simulink model "Microgrid_with_3VOCs"  (R2018a)
settings: Solver=VariableStepAuto  StartTime=0.0  StopTime=1  FixedStep=1e-4  MaxStep=1e-4  RelTol=1e-3
values from neighbouring files (symbols this model uses):
  Cosc = (P * Qf) / (wosc * Vrms^2)    [EpsilonGrapher.m]
  del = dK * Vrms * sqrt(2)    [EpsilonGrapher.m]
  k = double(Ms / zsysSupr)    [EpsilonGrapher.m]
  Lnet = (Vrms^2 * Lnpu) / (P * wosc)    (= 0.0198943678865)    [EpsilonGrapher.m]
  Losc = Vrms^2 / (wosc * P * Qf)    [EpsilonGrapher.m]
  Rnet = (Vrms^2 * Rnpu) / P    (= 6.25)    [EpsilonGrapher.m]
  Rosc = Vrms^2 / P    (= 62.5)    [EpsilonGrapher.m]
  Vrms = 250    [EpsilonGrapher.m]
undefined symbols (not defined in the file or in its folder): A, Continuous, fosc, gcbh, LIBRARY__Improved_VoC_with_DFs__2018_04_03__0, sps, sps_rtmsupport, spsMeanValueVariableFrequencyModel, spsPLLModel, VoC
libraries: powerlib x28, powerlib_meascontrol x13
settings Model: Creator=University  LastModifiedBy=rbtmc
settings SolverCC: ZeroCrossAlgorithm=Adaptive
settings DebuggingCC: MaxConsecutiveZCsMsg=none
settings CodeAppCC: StateflowObjectComments=on
settings SimscapeCC: SimscapeNormalizeSystem=off

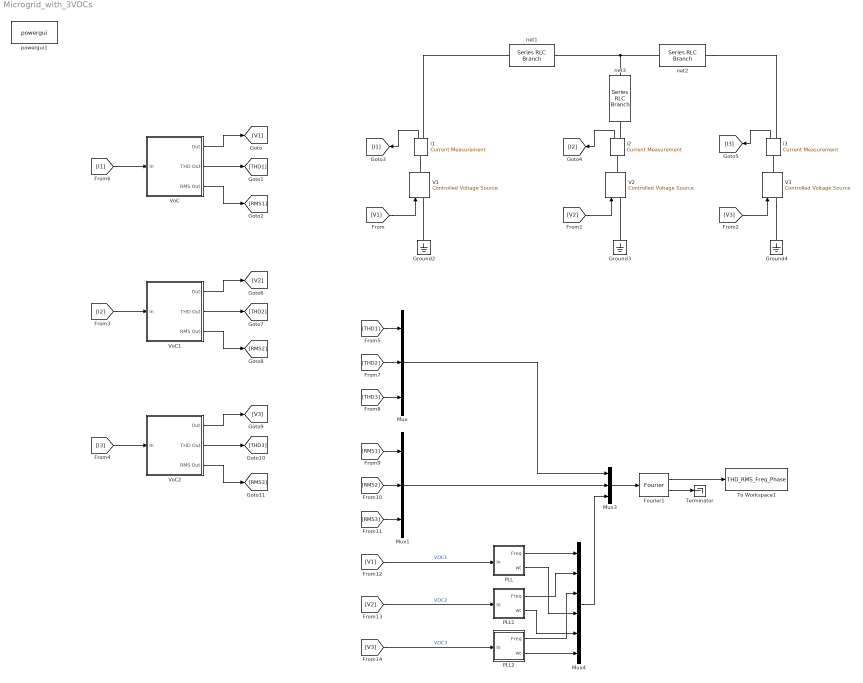
== system Microgrid_with_3VOCs ==
  Fourier1 : powerlib_meascontrol/Measurements/Fourier  Freq=50  n=0  InInit=[0, 0]  Ts=0
      settings: SourceProductName=Simscape Power Systems
  Ground2 : powerlib/Elements/Ground  LConnTagsString=a
  Ground3 : powerlib/Elements/Ground  LConnTagsString=a
  Ground4 : powerlib/Elements/Ground  LConnTagsString=a
  Mux : Mux  Inputs=3
  Mux1 : Mux  Inputs=3
  Mux3 : Mux  Inputs=3
  Mux4 : Mux  Inputs=6
  PLL : Subsystem  AncestorBlock=powerlib_meascontrol/PLL/PLL  DialogController=POWERSYS.PowerSysDialog  LoadFcn=sps_rtmsupport('LoadFcn', gcbh);  StartFcn=sps_rtmsupport('StartFcn', gcbh);  StopFcn=sps_rtmsupport('StopFcn', gcbh);  mask(PLL){Fmin=45, Par_Init=[0, 50], ParK=[180, 3200, 1], TcD=1e-4, MaxRateChangeFreq=12, FilterCutOffFreq=25, Ts=0, AGC=off}
      mask prompts: Fmin "Minimum frequency (Hz):"; Par_Init "Initial inputs [ Phase (degrees), Frequency (Hz) ]:"; ParK "Regulator gains [ Kp, Ki, Kd ]:"; TcD "Time constant for derivative action (s):"; MaxRateChangeFreq "Maximum rate of change of frequency (Hz/s):"; FilterCutOffFreq "Filter cut-off frequency for frequency measurement (Hz):"; Ts "Sample time:"; AGC "Enable automatic gain control"
      mask help:
      | This Phase Locked Loop (PLL) system can be used  to synchronize on a variable frequency sinusoidal signal. When the Automatic Gain Control is enabled, the input (phase error) of the PLL regulator is scaled according to the input signal magnitude.
      |
      | For optimal performance, set regulator gains [ Kp Ki  Kd ] = [ 180  3200  1 ] and check the Enable Automatic Gain Control parameter.
      |
      | Input : Normalized input signal (pu)
      | Output 1:  Measured frequency (Hz) = w/(2pi)
      | Output 2:  Ramp w.t varying between 0 and 2*pi, synchronized on the zero-crossing (rising) of the fundamental of input signal.
      mask init:
      | block=gcb;
      | [WantBlockChoice,Ts,sps] = powericon('PLLInit',block,Fmin,Par_Init,ParK,TcD,MaxRateChangeFreq,FilterCutOffFreq,AGC,Ts);
      | powericon('SetInternalModels','set',block,WantBlockChoice);
      settings: CopyFcn=sps_rtmsupport('CopyFcn', gcbh);  DeleteFcn=sps_rtmsupport('DeleteFcn', gcbh);  UndoDeleteFcn=sps_rtmsupport('UndoDeleteFcn', gcbh);  ModelCloseFcn=sps_rtmsupport('ModelCloseFcn', gcbh);  PreSaveFcn=sps_rtmsupport('PreSaveFcn', gcbh);  PostSaveFcn=sps_rtmsupport('PostSaveFcn', gcbh);  NameChangeFcn=sps_rtmsupport('NameChangeFcn', gcbh);  PreCopyFcn=sps_rtmsupport('PreCopyFcn', gcbh);  OpenFcn=sps_rtmsupport('OpenFcn', gcbh, [8]);  CloseFcn=sps_rtmsupport('CloseFcn', gcbh);  PreDeleteFcn=sps_rtmsupport('PreDeleteFcn', gcbh);
      mask Help: helpview(psbhelp);
  PLL1 : Subsystem  AncestorBlock=powerlib_meascontrol/PLL/PLL  DialogController=POWERSYS.PowerSysDialog  LoadFcn=sps_rtmsupport('LoadFcn', gcbh);  StartFcn=sps_rtmsupport('StartFcn', gcbh);  StopFcn=sps_rtmsupport('StopFcn', gcbh);  mask(PLL){Fmin=45, Par_Init=[0, 50], ParK=[180, 3200, 1], TcD=1e-4, MaxRateChangeFreq=12, FilterCutOffFreq=25, Ts=0, AGC=off}
      mask prompts: Fmin "Minimum frequency (Hz):"; Par_Init "Initial inputs [ Phase (degrees), Frequency (Hz) ]:"; ParK "Regulator gains [ Kp, Ki, Kd ]:"; TcD "Time constant for derivative action (s):"; MaxRateChangeFreq "Maximum rate of change of frequency (Hz/s):"; FilterCutOffFreq "Filter cut-off frequency for frequency measurement (Hz):"; Ts "Sample time:"; AGC "Enable automatic gain control"
      mask help:
      | This Phase Locked Loop (PLL) system can be used  to synchronize on a variable frequency sinusoidal signal. When the Automatic Gain Control is enabled, the input (phase error) of the PLL regulator is scaled according to the input signal magnitude.
      |
      | For optimal performance, set regulator gains [ Kp Ki  Kd ] = [ 180  3200  1 ] and check the Enable Automatic Gain Control parameter.
      |
      | Input : Normalized input signal (pu)
      | Output 1:  Measured frequency (Hz) = w/(2pi)
      | Output 2:  Ramp w.t varying between 0 and 2*pi, synchronized on the zero-crossing (rising) of the fundamental of input signal.
      mask init:
      | block=gcb;
      | [WantBlockChoice,Ts,sps] = powericon('PLLInit',block,Fmin,Par_Init,ParK,TcD,MaxRateChangeFreq,FilterCutOffFreq,AGC,Ts);
      | powericon('SetInternalModels','set',block,WantBlockChoice);
      settings: CopyFcn=sps_rtmsupport('CopyFcn', gcbh);  DeleteFcn=sps_rtmsupport('DeleteFcn', gcbh);  UndoDeleteFcn=sps_rtmsupport('UndoDeleteFcn', gcbh);  ModelCloseFcn=sps_rtmsupport('ModelCloseFcn', gcbh);  PreSaveFcn=sps_rtmsupport('PreSaveFcn', gcbh);  PostSaveFcn=sps_rtmsupport('PostSaveFcn', gcbh);  NameChangeFcn=sps_rtmsupport('NameChangeFcn', gcbh);  PreCopyFcn=sps_rtmsupport('PreCopyFcn', gcbh);  OpenFcn=sps_rtmsupport('OpenFcn', gcbh, [8]);  CloseFcn=sps_rtmsupport('CloseFcn', gcbh);  PreDeleteFcn=sps_rtmsupport('PreDeleteFcn', gcbh);
      mask Help: helpview(psbhelp);
  PLL2 : Subsystem  AncestorBlock=powerlib_meascontrol/PLL/PLL  DialogController=POWERSYS.PowerSysDialog  LoadFcn=sps_rtmsupport('LoadFcn', gcbh);  StartFcn=sps_rtmsupport('StartFcn', gcbh);  StopFcn=sps_rtmsupport('StopFcn', gcbh);  mask(PLL){Fmin=45, Par_Init=[0, 50], ParK=[180, 3200, 1], TcD=1e-4, MaxRateChangeFreq=12, FilterCutOffFreq=25, Ts=0, AGC=off}
      mask prompts: Fmin "Minimum frequency (Hz):"; Par_Init "Initial inputs [ Phase (degrees), Frequency (Hz) ]:"; ParK "Regulator gains [ Kp, Ki, Kd ]:"; TcD "Time constant for derivative action (s):"; MaxRateChangeFreq "Maximum rate of change of frequency (Hz/s):"; FilterCutOffFreq "Filter cut-off frequency for frequency measurement (Hz):"; Ts "Sample time:"; AGC "Enable automatic gain control"
      mask help:
      | This Phase Locked Loop (PLL) system can be used  to synchronize on a variable frequency sinusoidal signal. When the Automatic Gain Control is enabled, the input (phase error) of the PLL regulator is scaled according to the input signal magnitude.
      |
      | For optimal performance, set regulator gains [ Kp Ki  Kd ] = [ 180  3200  1 ] and check the Enable Automatic Gain Control parameter.
      |
      | Input : Normalized input signal (pu)
      | Output 1:  Measured frequency (Hz) = w/(2pi)
      | Output 2:  Ramp w.t varying between 0 and 2*pi, synchronized on the zero-crossing (rising) of the fundamental of input signal.
      mask init:
      | block=gcb;
      | [WantBlockChoice,Ts,sps] = powericon('PLLInit',block,Fmin,Par_Init,ParK,TcD,MaxRateChangeFreq,FilterCutOffFreq,AGC,Ts);
      | powericon('SetInternalModels','set',block,WantBlockChoice);
      settings: CopyFcn=sps_rtmsupport('CopyFcn', gcbh);  DeleteFcn=sps_rtmsupport('DeleteFcn', gcbh);  UndoDeleteFcn=sps_rtmsupport('UndoDeleteFcn', gcbh);  ModelCloseFcn=sps_rtmsupport('ModelCloseFcn', gcbh);  PreSaveFcn=sps_rtmsupport('PreSaveFcn', gcbh);  PostSaveFcn=sps_rtmsupport('PostSaveFcn', gcbh);  NameChangeFcn=sps_rtmsupport('NameChangeFcn', gcbh);  PreCopyFcn=sps_rtmsupport('PreCopyFcn', gcbh);  OpenFcn=sps_rtmsupport('OpenFcn', gcbh, [8]);  CloseFcn=sps_rtmsupport('CloseFcn', gcbh);  PreDeleteFcn=sps_rtmsupport('PreDeleteFcn', gcbh);
      mask Help: helpview(psbhelp);
  Terminator : Terminator
  To Workspace1 : ToWorkspace  VariableName=THD_RMS_Freq_Phase  SampleTime=-1
      settings: MaxDataPoints=1
  V1 : powerlib/Electrical Sources/Controlled Voltage Source  Initialize=off  Source_Type=AC  Amplitude=A  Phase=0  Frequency=fosc  Measurements=None
  V2 : powerlib/Electrical Sources/Controlled Voltage Source  Initialize=off  Source_Type=AC  Amplitude=A  Phase=120  Frequency=fosc  Measurements=None
  V3 : powerlib/Electrical Sources/Controlled Voltage Source  Initialize=off  Source_Type=AC  Amplitude=A  Phase=240  Frequency=fosc  Measurements=None
  VoC : Subsystem  AncestorBlock=LIBRARY__Improved_VoC_with_DFs__2018_04_03__0/VoC
  VoC1 : Subsystem  AncestorBlock=LIBRARY__Improved_VoC_with_DFs__2018_04_03__0/VoC
  VoC2 : Subsystem  AncestorBlock=LIBRARY__Improved_VoC_with_DFs__2018_04_03__0/VoC
  i1 : powerlib/Measurements/Current Measurement  PhasorSimulation=off  OutputType=Complex  PSBequivalent=0
  i2 : powerlib/Measurements/Current Measurement  PhasorSimulation=off  OutputType=Complex  PSBequivalent=0
  i3 : powerlib/Measurements/Current Measurement  PhasorSimulation=off  OutputType=Complex  PSBequivalent=0
  net1 : powerlib/Elements/Series RLC Branch  LConnTagsString=__new0  RConnTagsString=__new0  BranchType=RL  Resistance=Rnet  Inductance=Lnet  SetiL0=off  InitialCurrent=0  Capacitance=16.2e-3  Setx0=off  InitialVoltage=0  Measurements=None
  net2 : powerlib/Elements/Series RLC Branch  LConnTagsString=__new0  RConnTagsString=__new0  BranchType=RL  Resistance=Rnet  Inductance=Lnet  SetiL0=off  InitialCurrent=0  Capacitance=16.2e-3  Setx0=off  InitialVoltage=0  Measurements=None
  net3 : powerlib/Elements/Series RLC Branch  LConnTagsString=__new0  RConnTagsString=__new0  BranchType=RL  Resistance=Rnet  Inductance=Lnet  SetiL0=off  InitialCurrent=0  Capacitance=16.2e-3  Setx0=off  InitialVoltage=0  Measurements=None
  powergui1 : powerlib/powergui  Priority=1  SimulationMode=Discrete  SampleTime=50e-6  frequency=60  Iterations=50  frequencyindice=0  Pbase=100e6  ErrMax=1e-4  UnitsV=kV  UnitsW=MW  buscounter=0  FunctionMessages=off  echomessages=off  EnableUseOfTLC=off  CurrentSourceSwitches=off  DisableSnubberDevices=off  DisableRonSwitches=off  DisableVfSwitches=off  DisplayEquations=off  SolverType=Tustin/Backward Euler (TBE)  Interpol=off  ExternalGateDelay=off  methode=off  Ts=100  x0status=blocks  SPID=off  SwTol=0  HookPort=off  RestoreLinks=warning  ResistiveCurrentMeasurement=off  Frange=[0:2:500]  Ylog=off  Xlog=on  ShowGrid=off  save=off  variable=ZData  structure=0  ZoomFFT=off  StartTime=0.0  cycles=1  DisplayStyle=1  fundamental=60  FreqAxis=off  MaxFrequency=1000  frequencyindicesteady=1  RmsSteady=1  display=off
  wires:
  VoC/1(Out) -> [V1]
  VoC/2(THD Out) -> [THD1]
  VoC/3(RMS Out) -> [RMS1]
  [I1] -> VoC/1(In)
  i3/1 -> [I3]
  [V1] -> V1/1
  [V3] -> V3/1
  i2/1 -> [I2]
  i1/1 -> [I1]
  [V2] -> V2/1
  [I2] -> VoC1/1(In)
  VoC1/1(Out) -> [V2]
  VoC1/3(RMS Out) -> [RMS2]
  VoC1/2(THD Out) -> [THD2]
  [I3] -> VoC2/1(In)
  VoC2/1(Out) -> [V3]
  VoC2/3(RMS Out) -> [RMS3]
  VoC2/2(THD Out) -> [THD3]
  [THD1] -> Mux/1
  [THD2] -> Mux/2
  [THD3] -> Mux/3
  [RMS1] -> Mux1/1
  [RMS3] -> Mux1/3
  [RMS2] -> Mux1/2
  Mux/1 -> Mux3/1
  Mux1/1 -> Mux3/2
  [V1] -> PLL/1(In)  "VOC1"
  [V2] -> PLL1/1(In)  "VOC2"
  [V3] -> PLL2/1(In)  "VOC3"
  Mux3/1 -> Fourier1/1
  PLL/1(Freq) -> Mux4/1
  PLL1/1(Freq) -> Mux4/2
  PLL2/1(Freq) -> Mux4/3
  Mux4/1 -> Mux3/3
  Fourier1/1 -> To Workspace1/1
  PLL/2(wt) -> Mux4/4
  PLL1/2(wt) -> Mux4/5
  PLL2/2(wt) -> Mux4/6
  Fourier1/2 -> Terminator/1
  connections:
  i2/RConn1 -- net3/RConn1
  net1/RConn1 -- i1/RConn1
  i1/LConn1 -- V1/RConn1
  net2/RConn1 -- i3/RConn1
  V2/RConn1 -- i2/LConn1
  V3/LConn1 -- Ground4/LConn1
  V2/LConn1 -- Ground3/LConn1
  V3/RConn1 -- i3/LConn1
  Ground2/LConn1 -- V1/LConn1
  net3/LConn1 -- net2/LConn1 -- net1/LConn1

== system Microgrid_with_3VOCs/PLL ==
  In : Inport  SampleTime=Ts
  Model : Subsystem  AncestorBlock=spsPLLModel/Continuous  DialogController=POWERSYS.PowerSysDialog
  Freq : Outport  SampleTime=Ts
  wt : Outport  Port=2  SampleTime=Ts
  wires:
  Model/2(wt) -> wt/1
  Model/1(Freq) -> Freq/1
  In/1 -> Model/1(In)

== system Microgrid_with_3VOCs/PLL1 ==
  In : Inport  SampleTime=Ts
  Model : Subsystem  AncestorBlock=spsPLLModel/Continuous  DialogController=POWERSYS.PowerSysDialog
  Freq : Outport  SampleTime=Ts
  wt : Outport  Port=2  SampleTime=Ts
  wires:
  Model/2(wt) -> wt/1
  Model/1(Freq) -> Freq/1
  In/1 -> Model/1(In)

== system Microgrid_with_3VOCs/PLL2 ==
  In : Inport  SampleTime=Ts
  Model : Subsystem  AncestorBlock=spsPLLModel/Continuous  DialogController=POWERSYS.PowerSysDialog
  Freq : Outport  SampleTime=Ts
  wt : Outport  Port=2  SampleTime=Ts
  wires:
  Model/2(wt) -> wt/1
  Model/1(Freq) -> Freq/1
  In/1 -> Model/1(In)

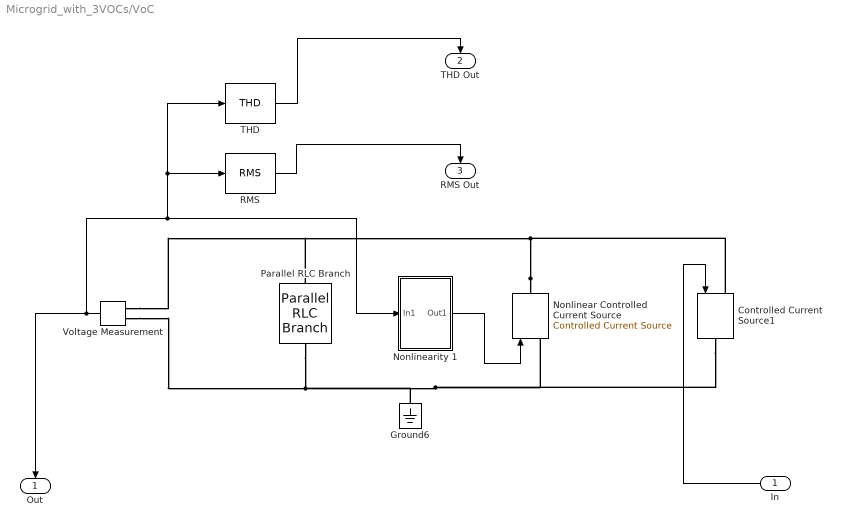
== system Microgrid_with_3VOCs/VoC ==
  In : Inport
  Controlled Current Source1 : powerlib/Electrical Sources/Controlled Current Source  Initialize=on  Source_Type=AC  Amplitude=0  Phase=0  Frequency=0  Measurements=None
  Ground6 : powerlib/Elements/Ground  LConnTagsString=a
  Nonlinear Controlled Current Source : powerlib/Electrical Sources/Controlled Current Source  Initialize=on  Source_Type=AC  Amplitude=0  Phase=0  Frequency=0  Measurements=None
  Nonlinearity 1 : Subsystem
  Parallel RLC Branch : powerlib/Elements/Parallel RLC Branch  LConnTagsString=a  RConnTagsString=__new0  BranchType=RLC  Resistance=Rosc  Inductance=Losc  SetiL0=off  InitialCurrent=0  Capacitance=Cosc  Setx0=on  InitialVoltage=Vrms * sqrt(2) * sind(0)  Measurements=None
  RMS : powerlib_meascontrol/Measurements/RMS  TrueRMS=on  Freq=50  RMSInit=0  Ts=0
  THD : powerlib_meascontrol/Measurements/THD  Freq=50  Ts=0
  Voltage Measurement : powerlib/Measurements/Voltage Measurement  PhasorSimulation=off  OutputType=Complex  PSBequivalent=0
  Out : Outport
  THD Out : Outport  Port=2
  RMS Out : Outport  Port=3
  wires:
  Voltage Measurement/1 -> THD/1, RMS/1, Nonlinearity 1/1(In1), Out/1
  In/1 -> Controlled Current Source1/1
  THD/1 -> THD Out/1
  RMS/1 -> RMS Out/1
  Nonlinearity 1/1(Out1) -> Nonlinear Controlled Current Source/1
  connections:
  Voltage Measurement/LConn2 -- Nonlinear Controlled Current Source/LConn1 -- Controlled Current Source1/RConn1 -- Ground6/LConn1 -- Parallel RLC Branch/RConn1
  Nonlinear Controlled Current Source/RConn1 -- Controlled Current Source1/LConn1 -- Voltage Measurement/LConn1 -- Parallel RLC Branch/LConn1

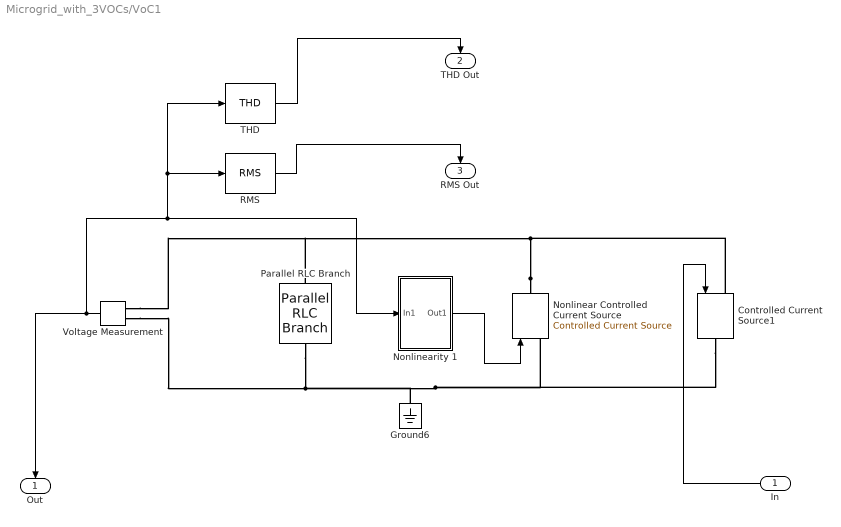
== system Microgrid_with_3VOCs/VoC1 ==
  In : Inport
  Controlled Current Source1 : powerlib/Electrical Sources/Controlled Current Source  Initialize=on  Source_Type=AC  Amplitude=0  Phase=0  Frequency=0  Measurements=None
  Ground6 : powerlib/Elements/Ground  LConnTagsString=a
  Nonlinear Controlled Current Source : powerlib/Electrical Sources/Controlled Current Source  Initialize=on  Source_Type=AC  Amplitude=0  Phase=0  Frequency=0  Measurements=None
  Nonlinearity 1 : Subsystem
  Parallel RLC Branch : powerlib/Elements/Parallel RLC Branch  LConnTagsString=a  RConnTagsString=__new0  BranchType=RLC  Resistance=Rosc  Inductance=Losc  SetiL0=off  InitialCurrent=0  Capacitance=Cosc  Setx0=on  InitialVoltage=Vrms * sqrt(2) * sind(45)  Measurements=None
  RMS : powerlib_meascontrol/Measurements/RMS  TrueRMS=on  Freq=50  RMSInit=0  Ts=0
  THD : powerlib_meascontrol/Measurements/THD  Freq=50  Ts=0
  Voltage Measurement : powerlib/Measurements/Voltage Measurement  PhasorSimulation=off  OutputType=Complex  PSBequivalent=0
  Out : Outport
  THD Out : Outport  Port=2
  RMS Out : Outport  Port=3
  wires:
  Voltage Measurement/1 -> THD/1, RMS/1, Nonlinearity 1/1(In1), Out/1
  In/1 -> Controlled Current Source1/1
  THD/1 -> THD Out/1
  RMS/1 -> RMS Out/1
  Nonlinearity 1/1(Out1) -> Nonlinear Controlled Current Source/1
  connections:
  Voltage Measurement/LConn2 -- Nonlinear Controlled Current Source/LConn1 -- Controlled Current Source1/RConn1 -- Ground6/LConn1 -- Parallel RLC Branch/RConn1
  Nonlinear Controlled Current Source/RConn1 -- Controlled Current Source1/LConn1 -- Voltage Measurement/LConn1 -- Parallel RLC Branch/LConn1

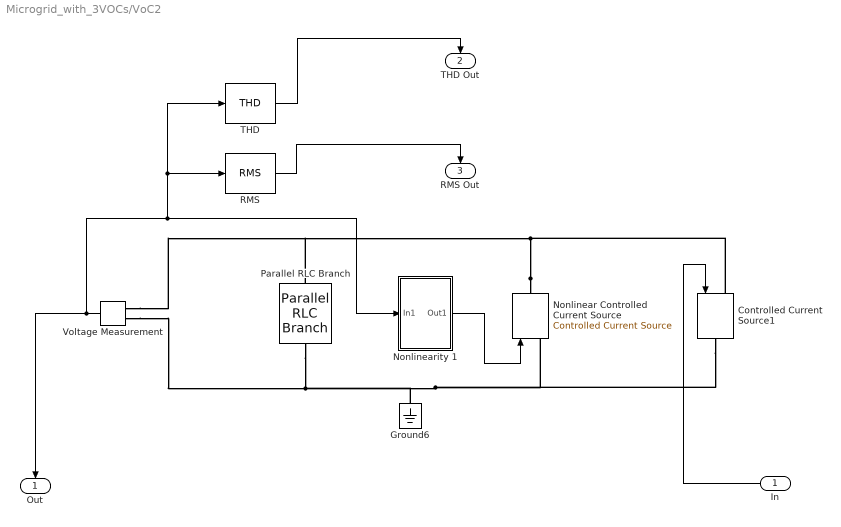
== system Microgrid_with_3VOCs/VoC2 ==
  In : Inport
  Controlled Current Source1 : powerlib/Electrical Sources/Controlled Current Source  Initialize=on  Source_Type=AC  Amplitude=0  Phase=0  Frequency=0  Measurements=None
  Ground6 : powerlib/Elements/Ground  LConnTagsString=a
  Nonlinear Controlled Current Source : powerlib/Electrical Sources/Controlled Current Source  Initialize=on  Source_Type=AC  Amplitude=0  Phase=0  Frequency=0  Measurements=None
  Nonlinearity 1 : Subsystem
  Parallel RLC Branch : powerlib/Elements/Parallel RLC Branch  LConnTagsString=a  RConnTagsString=__new0  BranchType=RLC  Resistance=Rosc  Inductance=Losc  SetiL0=off  InitialCurrent=0  Capacitance=Cosc  Setx0=on  InitialVoltage=Vrms * sqrt(2) * sind(90)  Measurements=None
  RMS : powerlib_meascontrol/Measurements/RMS  TrueRMS=on  Freq=50  RMSInit=0  Ts=0
  THD : powerlib_meascontrol/Measurements/THD  Freq=50  Ts=0
  Voltage Measurement : powerlib/Measurements/Voltage Measurement  PhasorSimulation=off  OutputType=Complex  PSBequivalent=0
  Out : Outport
  THD Out : Outport  Port=2
  RMS Out : Outport  Port=3
  wires:
  Voltage Measurement/1 -> THD/1, RMS/1, Nonlinearity 1/1(In1), Out/1
  In/1 -> Controlled Current Source1/1
  THD/1 -> THD Out/1
  RMS/1 -> RMS Out/1
  Nonlinearity 1/1(Out1) -> Nonlinear Controlled Current Source/1
  connections:
  Voltage Measurement/LConn2 -- Nonlinear Controlled Current Source/LConn1 -- Controlled Current Source1/RConn1 -- Ground6/LConn1 -- Parallel RLC Branch/RConn1
  Nonlinear Controlled Current Source/RConn1 -- Controlled Current Source1/LConn1 -- Voltage Measurement/LConn1 -- Parallel RLC Branch/LConn1

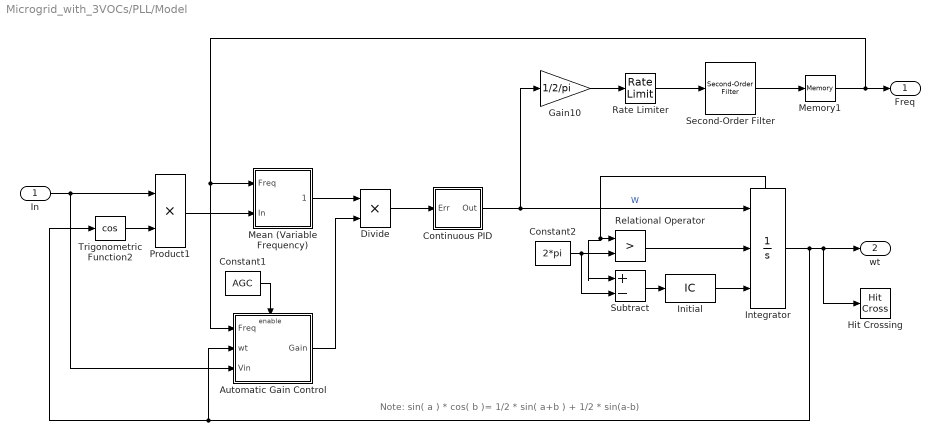
== system Microgrid_with_3VOCs/PLL/Model ==
  note: Note: sin( a ) * cos( b )= 1/2 * sin( a+b ) + 1/2 * sin(a-b)
  In : Inport
  Automatic Gain Control : Subsystem
  Constant1 : Constant  Value=AGC
  Constant2 : Constant  Value=2*pi
  Continuous PID : Subsystem  DialogController=POWERSYS.PowerSysDialog  VariantControl=PID_Continuous  mask(Continuous PID Controller){Kp=sps.Kp, Ki=sps.Ki, Kd=sps.Kd, TcD=sps.TcD, Par_Limits=[ inf  0 ], Init=2*pi*sps.Finit}
      mask prompts: Kp "Proportional gain (Kp):"; Ki "Integral gain (Ki):"; Kd "Derivative gain (Kd):"; TcD "Time constant for derivative filter (s):"; Par_Limits "Output limits: [ Upper   Lower ]"; Init "Output initial value:"
      mask help: This block implements a continuous PID controller.
      mask Display: disp('PID');
  Divide : Product
  Gain10 : Gain  Gain=1/2/pi  SaturateOnIntegerOverflow=on  OutDataTypeStr=Inherit: Same as input  ParamDataTypeStr=Inherit: Same as input
  Hit Crossing : HitCross  HitCrossingOffset=pi  HitCrossingDirection=falling  ShowOutputPort=off
  Initial : InitialCondition  Value=0
  Integrator : Integrator  ExternalReset=rising  InitialConditionSource=external  InitialCondition=sps.Phase_Init*pi/180  ShowStatePort=on
  Mean (Variable Frequency) : Subsystem  AncestorBlock=|  DialogController=POWERSYS.PowerSysDialog  LoadFcn=sps_rtmsupport('LoadFcn', gcbh);  StartFcn=sps_rtmsupport('StartFcn', gcbh);  StopFcn=sps_rtmsupport('StopFcn', gcbh);  mask(Mean (Variable Frequency)){Finit=sps.Finit, Fmin=sps.Fmin, Vinit=0, Ts=0}
      | powerlib_meascontrol/Measurements/Mean
      | (Variable Frequency)
      mask prompts: Finit "Initial frequency (Hz):"; Fmin "Minimum frequency (Hz):"; Vinit "Initial input (DC component):"; Ts "Sample time:"
      mask help:
      | Compute the mean value of input 2 over a running window of one cycle of frequency signal given by input 1.
      |
      | For the first cycle of initial frequency, the output is held to the value specified in the Initial input (DC component) parameter.
      |
      | The Minimum frequency parameter is used to determine the buffer size of the Variable Time Delay block used under the mask of the block.
      mask init:
      | block=gcb;
      | [WantBlockChoice,Ts,sps] = powericon('MeanVariableFrequencyInit',block,Finit,Fmin,Vinit,Ts);
      | powericon('SetInternalModels','set',block,WantBlockChoice);
      settings: CopyFcn=sps_rtmsupport('CopyFcn', gcbh);  DeleteFcn=sps_rtmsupport('DeleteFcn', gcbh);  UndoDeleteFcn=sps_rtmsupport('UndoDeleteFcn', gcbh);  ModelCloseFcn=sps_rtmsupport('ModelCloseFcn', gcbh);  PreSaveFcn=sps_rtmsupport('PreSaveFcn', gcbh);  PostSaveFcn=sps_rtmsupport('PostSaveFcn', gcbh);  NameChangeFcn=sps_rtmsupport('NameChangeFcn', gcbh);  PreCopyFcn=sps_rtmsupport('PreCopyFcn', gcbh);  OpenFcn=sps_rtmsupport('OpenFcn', gcbh, []);  CloseFcn=sps_rtmsupport('CloseFcn', gcbh);  PreDeleteFcn=sps_rtmsupport('PreDeleteFcn', gcbh);
      mask Help: helpview(psbhelp);
      mask Display:
      | port_label('input',1,'Freq')
      | port_label('input',2,'In')
      | plot(0,0, 1,1)
      | plot([0.8 1], [0.75 0.75])
      | plot([0.85 .95], [0.35 0.65],[0.85 .95], [0.65 0.35])
  Memory1 : Memory  InitialCondition=sps.Finit
  Product1 : Product  SaturateOnIntegerOverflow=on  InputSameDT=on  OutDataTypeStr=Inherit: Same as first input
  Rate Limiter : RateLimiter  RisingSlewLimit=sps.MaxRateChangeFreq  FallingSlewLimit=-sps.MaxRateChangeFreq  SampleTimeMode=inherited  InitialCondition=sps.Finit
  Relational Operator : RelationalOperator  Operator=>  OutDataTypeStr=boolean  RndMeth=Nearest
  Second-Order Filter : powerlib_meascontrol/Filters/Second-Order Filter  FilterType=Lowpass  Fo=sps.FilterCutOffFreq  Zeta=0.707  Ts=0  Initialize=on  Vac_Init=[0 0 sps.Finit]  Vdc_Init=sps.Finit  PlotResponse=off  FreqRange=[1 500 1]
      settings: SourceProductName=Simscape Power Systems  SourceProductBaseCode=PS
  Subtract : Sum  Inputs=+-
  Trigonometric Function2 : Trigonometry  Operator=cos
  Freq : Outport
  wt : Outport  Port=2
  wires:
  Initial/1 -> Integrator/3
  Subtract/1 -> Initial/1
  Integrator/State -> Subtract/1, Relational Operator/1
  Relational Operator/1 -> Integrator/2
  Constant2/1 -> Relational Operator/2, Subtract/2
  Trigonometric Function2/1 -> Product1/2
  Divide/1 -> Continuous PID/1(Err)
  Mean (Variable Frequency)/1(Mean) -> Divide/1
  Continuous PID/1(Out) -> Gain10/1, Integrator/1  "W"
  In/1 -> Automatic Gain Control/3(Vin), Product1/1
  Integrator/1 -> Automatic Gain Control/2(wt), Trigonometric Function2/1, Hit Crossing/1, wt/1
  Gain10/1 -> Rate Limiter/1
  Rate Limiter/1 -> Second-Order Filter/1
  Second-Order Filter/1 -> Memory1/1
  Product1/1 -> Mean (Variable Frequency)/2(In)
  Constant1/1 -> Automatic Gain Control/Enable
  Automatic Gain Control/1(Gain) -> Divide/2
  Memory1/1 -> Freq/1, Mean (Variable Frequency)/1(Freq), Automatic Gain Control/1(Freq)

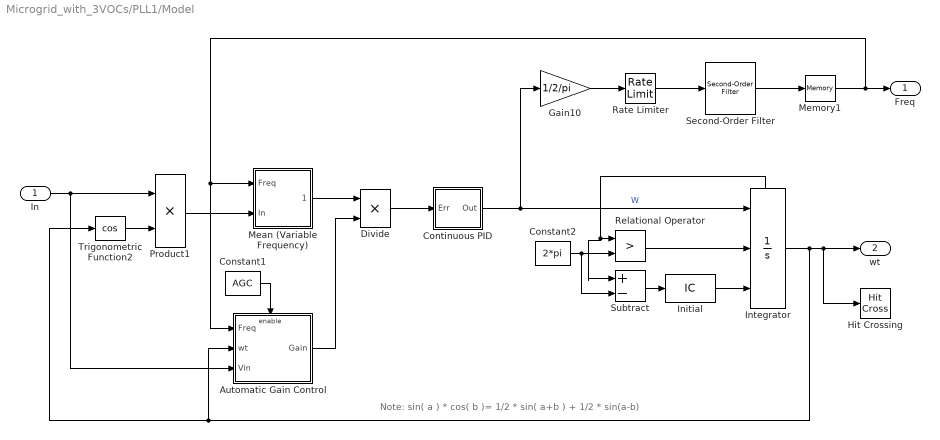
== system Microgrid_with_3VOCs/PLL1/Model ==
  note: Note: sin( a ) * cos( b )= 1/2 * sin( a+b ) + 1/2 * sin(a-b)
  In : Inport
  Automatic Gain Control : Subsystem
  Constant1 : Constant  Value=AGC
  Constant2 : Constant  Value=2*pi
  Continuous PID : Subsystem  DialogController=POWERSYS.PowerSysDialog  VariantControl=PID_Continuous  mask(Continuous PID Controller){Kp=sps.Kp, Ki=sps.Ki, Kd=sps.Kd, TcD=sps.TcD, Par_Limits=[ inf  0 ], Init=2*pi*sps.Finit}
      mask prompts: Kp "Proportional gain (Kp):"; Ki "Integral gain (Ki):"; Kd "Derivative gain (Kd):"; TcD "Time constant for derivative filter (s):"; Par_Limits "Output limits: [ Upper   Lower ]"; Init "Output initial value:"
      mask help: This block implements a continuous PID controller.
      mask Display: disp('PID');
  Divide : Product
  Gain10 : Gain  Gain=1/2/pi  SaturateOnIntegerOverflow=on  OutDataTypeStr=Inherit: Same as input  ParamDataTypeStr=Inherit: Same as input
  Hit Crossing : HitCross  HitCrossingOffset=pi  HitCrossingDirection=falling  ShowOutputPort=off
  Initial : InitialCondition  Value=0
  Integrator : Integrator  ExternalReset=rising  InitialConditionSource=external  InitialCondition=sps.Phase_Init*pi/180  ShowStatePort=on
  Mean (Variable Frequency) : Subsystem  AncestorBlock=|  DialogController=POWERSYS.PowerSysDialog  LoadFcn=sps_rtmsupport('LoadFcn', gcbh);  StartFcn=sps_rtmsupport('StartFcn', gcbh);  StopFcn=sps_rtmsupport('StopFcn', gcbh);  mask(Mean (Variable Frequency)){Finit=sps.Finit, Fmin=sps.Fmin, Vinit=0, Ts=0}
      | powerlib_meascontrol/Measurements/Mean
      | (Variable Frequency)
      mask prompts: Finit "Initial frequency (Hz):"; Fmin "Minimum frequency (Hz):"; Vinit "Initial input (DC component):"; Ts "Sample time:"
      mask help:
      | Compute the mean value of input 2 over a running window of one cycle of frequency signal given by input 1.
      |
      | For the first cycle of initial frequency, the output is held to the value specified in the Initial input (DC component) parameter.
      |
      | The Minimum frequency parameter is used to determine the buffer size of the Variable Time Delay block used under the mask of the block.
      mask init:
      | block=gcb;
      | [WantBlockChoice,Ts,sps] = powericon('MeanVariableFrequencyInit',block,Finit,Fmin,Vinit,Ts);
      | powericon('SetInternalModels','set',block,WantBlockChoice);
      settings: CopyFcn=sps_rtmsupport('CopyFcn', gcbh);  DeleteFcn=sps_rtmsupport('DeleteFcn', gcbh);  UndoDeleteFcn=sps_rtmsupport('UndoDeleteFcn', gcbh);  ModelCloseFcn=sps_rtmsupport('ModelCloseFcn', gcbh);  PreSaveFcn=sps_rtmsupport('PreSaveFcn', gcbh);  PostSaveFcn=sps_rtmsupport('PostSaveFcn', gcbh);  NameChangeFcn=sps_rtmsupport('NameChangeFcn', gcbh);  PreCopyFcn=sps_rtmsupport('PreCopyFcn', gcbh);  OpenFcn=sps_rtmsupport('OpenFcn', gcbh, []);  CloseFcn=sps_rtmsupport('CloseFcn', gcbh);  PreDeleteFcn=sps_rtmsupport('PreDeleteFcn', gcbh);
      mask Help: helpview(psbhelp);
      mask Display:
      | port_label('input',1,'Freq')
      | port_label('input',2,'In')
      | plot(0,0, 1,1)
      | plot([0.8 1], [0.75 0.75])
      | plot([0.85 .95], [0.35 0.65],[0.85 .95], [0.65 0.35])
  Memory1 : Memory  InitialCondition=sps.Finit
  Product1 : Product  SaturateOnIntegerOverflow=on  InputSameDT=on  OutDataTypeStr=Inherit: Same as first input
  Rate Limiter : RateLimiter  RisingSlewLimit=sps.MaxRateChangeFreq  FallingSlewLimit=-sps.MaxRateChangeFreq  SampleTimeMode=inherited  InitialCondition=sps.Finit
  Relational Operator : RelationalOperator  Operator=>  OutDataTypeStr=boolean  RndMeth=Nearest
  Second-Order Filter : powerlib_meascontrol/Filters/Second-Order Filter  FilterType=Lowpass  Fo=sps.FilterCutOffFreq  Zeta=0.707  Ts=0  Initialize=on  Vac_Init=[0 0 sps.Finit]  Vdc_Init=sps.Finit  PlotResponse=off  FreqRange=[1 500 1]
      settings: SourceProductName=Simscape Power Systems  SourceProductBaseCode=PS
  Subtract : Sum  Inputs=+-
  Trigonometric Function2 : Trigonometry  Operator=cos
  Freq : Outport
  wt : Outport  Port=2
  wires:
  Initial/1 -> Integrator/3
  Subtract/1 -> Initial/1
  Integrator/State -> Subtract/1, Relational Operator/1
  Relational Operator/1 -> Integrator/2
  Constant2/1 -> Relational Operator/2, Subtract/2
  Trigonometric Function2/1 -> Product1/2
  Divide/1 -> Continuous PID/1(Err)
  Mean (Variable Frequency)/1(Mean) -> Divide/1
  Continuous PID/1(Out) -> Gain10/1, Integrator/1  "W"
  In/1 -> Automatic Gain Control/3(Vin), Product1/1
  Integrator/1 -> Automatic Gain Control/2(wt), Trigonometric Function2/1, Hit Crossing/1, wt/1
  Gain10/1 -> Rate Limiter/1
  Rate Limiter/1 -> Second-Order Filter/1
  Second-Order Filter/1 -> Memory1/1
  Product1/1 -> Mean (Variable Frequency)/2(In)
  Constant1/1 -> Automatic Gain Control/Enable
  Automatic Gain Control/1(Gain) -> Divide/2
  Memory1/1 -> Freq/1, Mean (Variable Frequency)/1(Freq), Automatic Gain Control/1(Freq)

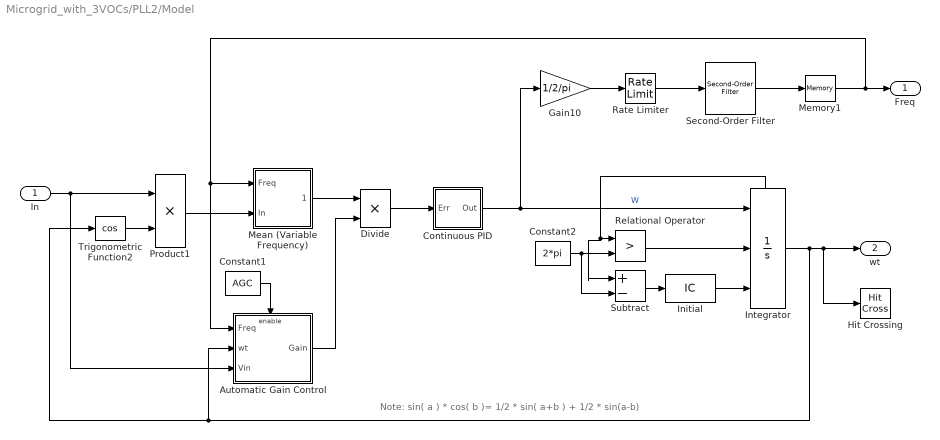
== system Microgrid_with_3VOCs/PLL2/Model ==
  note: Note: sin( a ) * cos( b )= 1/2 * sin( a+b ) + 1/2 * sin(a-b)
  In : Inport
  Automatic Gain Control : Subsystem
  Constant1 : Constant  Value=AGC
  Constant2 : Constant  Value=2*pi
  Continuous PID : Subsystem  DialogController=POWERSYS.PowerSysDialog  VariantControl=PID_Continuous  mask(Continuous PID Controller){Kp=sps.Kp, Ki=sps.Ki, Kd=sps.Kd, TcD=sps.TcD, Par_Limits=[ inf  0 ], Init=2*pi*sps.Finit}
      mask prompts: Kp "Proportional gain (Kp):"; Ki "Integral gain (Ki):"; Kd "Derivative gain (Kd):"; TcD "Time constant for derivative filter (s):"; Par_Limits "Output limits: [ Upper   Lower ]"; Init "Output initial value:"
      mask help: This block implements a continuous PID controller.
      mask Display: disp('PID');
  Divide : Product
  Gain10 : Gain  Gain=1/2/pi  SaturateOnIntegerOverflow=on  OutDataTypeStr=Inherit: Same as input  ParamDataTypeStr=Inherit: Same as input
  Hit Crossing : HitCross  HitCrossingOffset=pi  HitCrossingDirection=falling  ShowOutputPort=off
  Initial : InitialCondition  Value=0
  Integrator : Integrator  ExternalReset=rising  InitialConditionSource=external  InitialCondition=sps.Phase_Init*pi/180  ShowStatePort=on
  Mean (Variable Frequency) : Subsystem  AncestorBlock=|  DialogController=POWERSYS.PowerSysDialog  LoadFcn=sps_rtmsupport('LoadFcn', gcbh);  StartFcn=sps_rtmsupport('StartFcn', gcbh);  StopFcn=sps_rtmsupport('StopFcn', gcbh);  mask(Mean (Variable Frequency)){Finit=sps.Finit, Fmin=sps.Fmin, Vinit=0, Ts=0}
      | powerlib_meascontrol/Measurements/Mean
      | (Variable Frequency)
      mask prompts: Finit "Initial frequency (Hz):"; Fmin "Minimum frequency (Hz):"; Vinit "Initial input (DC component):"; Ts "Sample time:"
      mask help:
      | Compute the mean value of input 2 over a running window of one cycle of frequency signal given by input 1.
      |
      | For the first cycle of initial frequency, the output is held to the value specified in the Initial input (DC component) parameter.
      |
      | The Minimum frequency parameter is used to determine the buffer size of the Variable Time Delay block used under the mask of the block.
      mask init:
      | block=gcb;
      | [WantBlockChoice,Ts,sps] = powericon('MeanVariableFrequencyInit',block,Finit,Fmin,Vinit,Ts);
      | powericon('SetInternalModels','set',block,WantBlockChoice);
      settings: CopyFcn=sps_rtmsupport('CopyFcn', gcbh);  DeleteFcn=sps_rtmsupport('DeleteFcn', gcbh);  UndoDeleteFcn=sps_rtmsupport('UndoDeleteFcn', gcbh);  ModelCloseFcn=sps_rtmsupport('ModelCloseFcn', gcbh);  PreSaveFcn=sps_rtmsupport('PreSaveFcn', gcbh);  PostSaveFcn=sps_rtmsupport('PostSaveFcn', gcbh);  NameChangeFcn=sps_rtmsupport('NameChangeFcn', gcbh);  PreCopyFcn=sps_rtmsupport('PreCopyFcn', gcbh);  OpenFcn=sps_rtmsupport('OpenFcn', gcbh, []);  CloseFcn=sps_rtmsupport('CloseFcn', gcbh);  PreDeleteFcn=sps_rtmsupport('PreDeleteFcn', gcbh);
      mask Help: helpview(psbhelp);
      mask Display:
      | port_label('input',1,'Freq')
      | port_label('input',2,'In')
      | plot(0,0, 1,1)
      | plot([0.8 1], [0.75 0.75])
      | plot([0.85 .95], [0.35 0.65],[0.85 .95], [0.65 0.35])
  Memory1 : Memory  InitialCondition=sps.Finit
  Product1 : Product  SaturateOnIntegerOverflow=on  InputSameDT=on  OutDataTypeStr=Inherit: Same as first input
  Rate Limiter : RateLimiter  RisingSlewLimit=sps.MaxRateChangeFreq  FallingSlewLimit=-sps.MaxRateChangeFreq  SampleTimeMode=inherited  InitialCondition=sps.Finit
  Relational Operator : RelationalOperator  Operator=>  OutDataTypeStr=boolean  RndMeth=Nearest
  Second-Order Filter : powerlib_meascontrol/Filters/Second-Order Filter  FilterType=Lowpass  Fo=sps.FilterCutOffFreq  Zeta=0.707  Ts=0  Initialize=on  Vac_Init=[0 0 sps.Finit]  Vdc_Init=sps.Finit  PlotResponse=off  FreqRange=[1 500 1]
      settings: SourceProductName=Simscape Power Systems  SourceProductBaseCode=PS
  Subtract : Sum  Inputs=+-
  Trigonometric Function2 : Trigonometry  Operator=cos
  Freq : Outport
  wt : Outport  Port=2
  wires:
  Initial/1 -> Integrator/3
  Subtract/1 -> Initial/1
  Integrator/State -> Subtract/1, Relational Operator/1
  Relational Operator/1 -> Integrator/2
  Constant2/1 -> Relational Operator/2, Subtract/2
  Trigonometric Function2/1 -> Product1/2
  Divide/1 -> Continuous PID/1(Err)
  Mean (Variable Frequency)/1(Mean) -> Divide/1
  Continuous PID/1(Out) -> Gain10/1, Integrator/1  "W"
  In/1 -> Automatic Gain Control/3(Vin), Product1/1
  Integrator/1 -> Automatic Gain Control/2(wt), Trigonometric Function2/1, Hit Crossing/1, wt/1
  Gain10/1 -> Rate Limiter/1
  Rate Limiter/1 -> Second-Order Filter/1
  Second-Order Filter/1 -> Memory1/1
  Product1/1 -> Mean (Variable Frequency)/2(In)
  Constant1/1 -> Automatic Gain Control/Enable
  Automatic Gain Control/1(Gain) -> Divide/2
  Memory1/1 -> Freq/1, Mean (Variable Frequency)/1(Freq), Automatic Gain Control/1(Freq)

== system Microgrid_with_3VOCs/VoC/Nonlinearity 1 ==
  In1 : Inport
  MATLAB Function : MATLAB Function  TreatAsAtomicUnit=on
  Phi : Constant  Value=del
  Sig : Constant  Value=k
  Out1 : Outport
  wires:
  MATLAB Function/1(I) -> Out1/1
  In1/1 -> MATLAB Function/1(V)
  Phi/1 -> MATLAB Function/3(Phi)
  Sig/1 -> MATLAB Function/2(Sig)

== system Microgrid_with_3VOCs/VoC1/Nonlinearity 1 ==
  In1 : Inport
  MATLAB Function : MATLAB Function  TreatAsAtomicUnit=on
  Phi : Constant  Value=del
  Sig : Constant  Value=k
  Out1 : Outport
  wires:
  MATLAB Function/1(I) -> Out1/1
  In1/1 -> MATLAB Function/1(V)
  Phi/1 -> MATLAB Function/3(Phi)
  Sig/1 -> MATLAB Function/2(Sig)

== system Microgrid_with_3VOCs/VoC2/Nonlinearity 1 ==
  In1 : Inport
  MATLAB Function : MATLAB Function  TreatAsAtomicUnit=on
  Phi : Constant  Value=del
  Sig : Constant  Value=k
  Out1 : Outport
  wires:
  MATLAB Function/1(I) -> Out1/1
  In1/1 -> MATLAB Function/1(V)
  Phi/1 -> MATLAB Function/3(Phi)
  Sig/1 -> MATLAB Function/2(Sig)

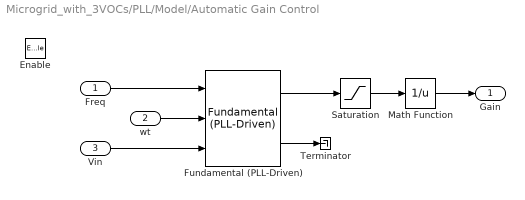
== system Microgrid_with_3VOCs/PLL/Model/Automatic Gain Control ==
  Freq : Inport
  wt : Inport  Port=2
  Vin : Inport  Port=3
  Enable : EnablePort  PropagateVarSize=During execution
  Fundamental (PLL-Driven) : powerlib_meascontrol/Measurements/Fundamental (PLL-Driven)  Finit=sps.Finit  Fmin=sps.Fmin  InInit=[1 sps.Phase_Init*pi/180]  Ts=0
      settings: SourceProductName=Simscape Power Systems  SourceProductBaseCode=PS
  Math Function : Math  Operator=reciprocal  SaturateOnIntegerOverflow=on
  Saturation : Saturate  UpperLimit=inf  LowerLimit=eps
  Terminator : Terminator
  Gain : Outport  InitialOutput=[1]
  wires:
  wt/1 -> Fundamental (PLL-Driven)/2
  Fundamental (PLL-Driven)/2 -> Terminator/1
  Saturation/1 -> Math Function/1
  Fundamental (PLL-Driven)/1 -> Saturation/1
  Freq/1 -> Fundamental (PLL-Driven)/1
  Vin/1 -> Fundamental (PLL-Driven)/3
  Math Function/1 -> Gain/1

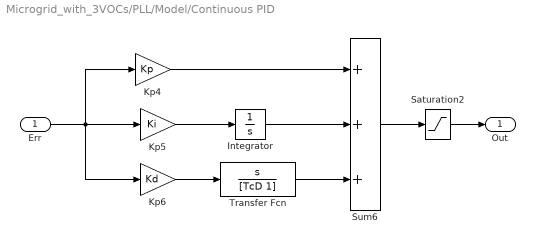
== system Microgrid_with_3VOCs/PLL/Model/Continuous PID ==
  Err : Inport  SampleTime=0
  Integrator : Integrator  InitialCondition=Init  LimitOutput=on  UpperSaturationLimit=Par_Limits(1)  LowerSaturationLimit=Par_Limits(2)
  Kp4 : Gain  Gain=Kp  SampleTime=0  SaturateOnIntegerOverflow=on  OutDataTypeStr=Inherit: Same as input  ParamDataTypeStr=Inherit: Same as input
  Kp5 : Gain  Gain=Ki  SampleTime=0  SaturateOnIntegerOverflow=on  OutDataTypeStr=Inherit: Same as input  ParamDataTypeStr=Inherit: Same as input
  Kp6 : Gain  Gain=Kd  SampleTime=0  SaturateOnIntegerOverflow=on  OutDataTypeStr=Inherit: Same as input  ParamDataTypeStr=Inherit: Same as input
  Saturation2 : Saturate  UpperLimit=Par_Limits(1)  LowerLimit=Par_Limits(2)  ZeroCross=off  SampleTime=0
  Sum6 : Sum  Inputs=+++  SampleTime=0  SaturateOnIntegerOverflow=on  InputSameDT=on  OutDataTypeStr=Inherit: Same as first input
  Transfer Fcn : TransferFcn  Numerator=[1 0]  Denominator=[TcD 1]
  Out : Outport  SampleTime=0  InitialOutput=0
  wires:
  Saturation2/1 -> Out/1
  Err/1 -> Kp4/1, Kp5/1, Kp6/1
  Sum6/1 -> Saturation2/1
  Kp5/1 -> Integrator/1
  Kp6/1 -> Transfer Fcn/1
  Kp4/1 -> Sum6/1
  Integrator/1 -> Sum6/2
  Transfer Fcn/1 -> Sum6/3

== system Microgrid_with_3VOCs/PLL/Model/Mean (Variable Frequency) ==
  Freq : Inport  PortDimensions=1  SampleTime=Ts
  In : Inport  Port=2  SampleTime=Ts
  Model : Subsystem  AncestorBlock=spsMeanValueVariableFrequencyModel/Continuous
  Mean : Outport  SampleTime=Ts
  wires:
  Model/1(Mean) -> Mean/1
  In/1 -> Model/2(In)
  Freq/1 -> Model/1(Freq)

== system Microgrid_with_3VOCs/PLL1/Model/Automatic Gain Control ==
  Freq : Inport
  wt : Inport  Port=2
  Vin : Inport  Port=3
  Enable : EnablePort  PropagateVarSize=During execution
  Fundamental (PLL-Driven) : powerlib_meascontrol/Measurements/Fundamental (PLL-Driven)  Finit=sps.Finit  Fmin=sps.Fmin  InInit=[1 sps.Phase_Init*pi/180]  Ts=0
      settings: SourceProductName=Simscape Power Systems  SourceProductBaseCode=PS
  Math Function : Math  Operator=reciprocal  SaturateOnIntegerOverflow=on
  Saturation : Saturate  UpperLimit=inf  LowerLimit=eps
  Terminator : Terminator
  Gain : Outport  InitialOutput=[1]
  wires:
  wt/1 -> Fundamental (PLL-Driven)/2
  Fundamental (PLL-Driven)/2 -> Terminator/1
  Saturation/1 -> Math Function/1
  Fundamental (PLL-Driven)/1 -> Saturation/1
  Freq/1 -> Fundamental (PLL-Driven)/1
  Vin/1 -> Fundamental (PLL-Driven)/3
  Math Function/1 -> Gain/1

== system Microgrid_with_3VOCs/PLL1/Model/Continuous PID ==
  Err : Inport  SampleTime=0
  Integrator : Integrator  InitialCondition=Init  LimitOutput=on  UpperSaturationLimit=Par_Limits(1)  LowerSaturationLimit=Par_Limits(2)
  Kp4 : Gain  Gain=Kp  SampleTime=0  SaturateOnIntegerOverflow=on  OutDataTypeStr=Inherit: Same as input  ParamDataTypeStr=Inherit: Same as input
  Kp5 : Gain  Gain=Ki  SampleTime=0  SaturateOnIntegerOverflow=on  OutDataTypeStr=Inherit: Same as input  ParamDataTypeStr=Inherit: Same as input
  Kp6 : Gain  Gain=Kd  SampleTime=0  SaturateOnIntegerOverflow=on  OutDataTypeStr=Inherit: Same as input  ParamDataTypeStr=Inherit: Same as input
  Saturation2 : Saturate  UpperLimit=Par_Limits(1)  LowerLimit=Par_Limits(2)  ZeroCross=off  SampleTime=0
  Sum6 : Sum  Inputs=+++  SampleTime=0  SaturateOnIntegerOverflow=on  InputSameDT=on  OutDataTypeStr=Inherit: Same as first input
  Transfer Fcn : TransferFcn  Numerator=[1 0]  Denominator=[TcD 1]
  Out : Outport  SampleTime=0  InitialOutput=0
  wires:
  Saturation2/1 -> Out/1
  Err/1 -> Kp4/1, Kp5/1, Kp6/1
  Sum6/1 -> Saturation2/1
  Kp5/1 -> Integrator/1
  Kp6/1 -> Transfer Fcn/1
  Kp4/1 -> Sum6/1
  Integrator/1 -> Sum6/2
  Transfer Fcn/1 -> Sum6/3

== system Microgrid_with_3VOCs/PLL1/Model/Mean (Variable Frequency) ==
  Freq : Inport  PortDimensions=1  SampleTime=Ts
  In : Inport  Port=2  SampleTime=Ts
  Model : Subsystem  AncestorBlock=spsMeanValueVariableFrequencyModel/Continuous
  Mean : Outport  SampleTime=Ts
  wires:
  Model/1(Mean) -> Mean/1
  In/1 -> Model/2(In)
  Freq/1 -> Model/1(Freq)

== system Microgrid_with_3VOCs/PLL2/Model/Automatic Gain Control ==
  Freq : Inport
  wt : Inport  Port=2
  Vin : Inport  Port=3
  Enable : EnablePort  PropagateVarSize=During execution
  Fundamental (PLL-Driven) : powerlib_meascontrol/Measurements/Fundamental (PLL-Driven)  Finit=sps.Finit  Fmin=sps.Fmin  InInit=[1 sps.Phase_Init*pi/180]  Ts=0
      settings: SourceProductName=Simscape Power Systems  SourceProductBaseCode=PS
  Math Function : Math  Operator=reciprocal  SaturateOnIntegerOverflow=on
  Saturation : Saturate  UpperLimit=inf  LowerLimit=eps
  Terminator : Terminator
  Gain : Outport  InitialOutput=[1]
  wires:
  wt/1 -> Fundamental (PLL-Driven)/2
  Fundamental (PLL-Driven)/2 -> Terminator/1
  Saturation/1 -> Math Function/1
  Fundamental (PLL-Driven)/1 -> Saturation/1
  Freq/1 -> Fundamental (PLL-Driven)/1
  Vin/1 -> Fundamental (PLL-Driven)/3
  Math Function/1 -> Gain/1

== system Microgrid_with_3VOCs/PLL2/Model/Continuous PID ==
  Err : Inport  SampleTime=0
  Integrator : Integrator  InitialCondition=Init  LimitOutput=on  UpperSaturationLimit=Par_Limits(1)  LowerSaturationLimit=Par_Limits(2)
  Kp4 : Gain  Gain=Kp  SampleTime=0  SaturateOnIntegerOverflow=on  OutDataTypeStr=Inherit: Same as input  ParamDataTypeStr=Inherit: Same as input
  Kp5 : Gain  Gain=Ki  SampleTime=0  SaturateOnIntegerOverflow=on  OutDataTypeStr=Inherit: Same as input  ParamDataTypeStr=Inherit: Same as input
  Kp6 : Gain  Gain=Kd  SampleTime=0  SaturateOnIntegerOverflow=on  OutDataTypeStr=Inherit: Same as input  ParamDataTypeStr=Inherit: Same as input
  Saturation2 : Saturate  UpperLimit=Par_Limits(1)  LowerLimit=Par_Limits(2)  ZeroCross=off  SampleTime=0
  Sum6 : Sum  Inputs=+++  SampleTime=0  SaturateOnIntegerOverflow=on  InputSameDT=on  OutDataTypeStr=Inherit: Same as first input
  Transfer Fcn : TransferFcn  Numerator=[1 0]  Denominator=[TcD 1]
  Out : Outport  SampleTime=0  InitialOutput=0
  wires:
  Saturation2/1 -> Out/1
  Err/1 -> Kp4/1, Kp5/1, Kp6/1
  Sum6/1 -> Saturation2/1
  Kp5/1 -> Integrator/1
  Kp6/1 -> Transfer Fcn/1
  Kp4/1 -> Sum6/1
  Integrator/1 -> Sum6/2
  Transfer Fcn/1 -> Sum6/3

== system Microgrid_with_3VOCs/PLL2/Model/Mean (Variable Frequency) ==
  Freq : Inport  PortDimensions=1  SampleTime=Ts
  In : Inport  Port=2  SampleTime=Ts
  Model : Subsystem  AncestorBlock=spsMeanValueVariableFrequencyModel/Continuous
  Mean : Outport  SampleTime=Ts
  wires:
  Model/1(Mean) -> Mean/1
  In/1 -> Model/2(In)
  Freq/1 -> Model/1(Freq)

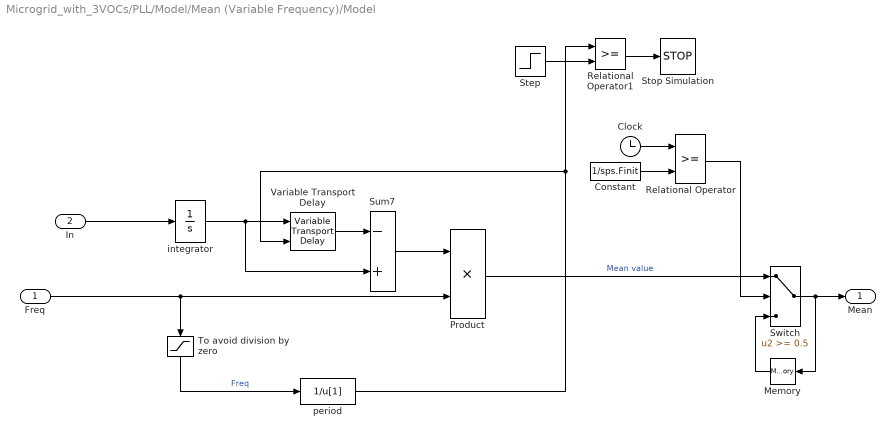
== system Microgrid_with_3VOCs/PLL/Model/Mean (Variable Frequency)/Model ==
  Freq : Inport  PortDimensions=1
  In : Inport  Port=2
  Clock : Clock
  Constant : Constant  Value=1/sps.Finit
  Memory : Memory  InitialCondition=sps.Vinit
  Product : Product  SaturateOnIntegerOverflow=on  InputSameDT=on  OutDataTypeStr=Inherit: Same as first input
  Relational Operator : RelationalOperator  OutDataTypeStr=boolean  SampleTime=Ts  RndMeth=Nearest
  Relational Operator1 : RelationalOperator  OutDataTypeStr=boolean  RndMeth=Simplest
  Step : Step  Time=0.1  Before=10e6  After=0.016  SampleTime=0
  Stop Simulation : Stop
  Sum7 : Sum  Inputs=-+  SaturateOnIntegerOverflow=on  InputSameDT=on  OutDataTypeStr=Inherit: Same as first input
  Switch : Switch  Threshold=0.5  InputSameDT=on
  To avoid division by zero : Saturate  UpperLimit=1e6  LowerLimit=eps
  Variable Transport Delay : VariableTransportDelay  VariableDelayType=Variable transport delay  MaximumDelay=1/sps.Fmin+eps  MaximumPoints=2048*4  PadeOrder=2
  integrator : Integrator
  period : Fcn  Expr=1/u[1]
  Mean : Outport
  wires:
  Constant/1 -> Relational Operator/2
  To avoid division by zero/1 -> period/1  "Freq"
  Switch/1 -> Memory/1, Mean/1
  Freq/1 -> To avoid division by zero/1, Product/2
  integrator/1 -> Variable Transport Delay/1, Sum7/2
  Sum7/1 -> Product/1
  Variable Transport Delay/1 -> Sum7/1
  Product/1 -> Switch/1  "Mean value"
  In/1 -> integrator/1
  Clock/1 -> Relational Operator/1
  Memory/1 -> Switch/3
  Relational Operator/1 -> Switch/2
  Relational Operator1/1 -> Stop Simulation/1
  Step/1 -> Relational Operator1/2
  period/1 -> Variable Transport Delay/2, Relational Operator1/1

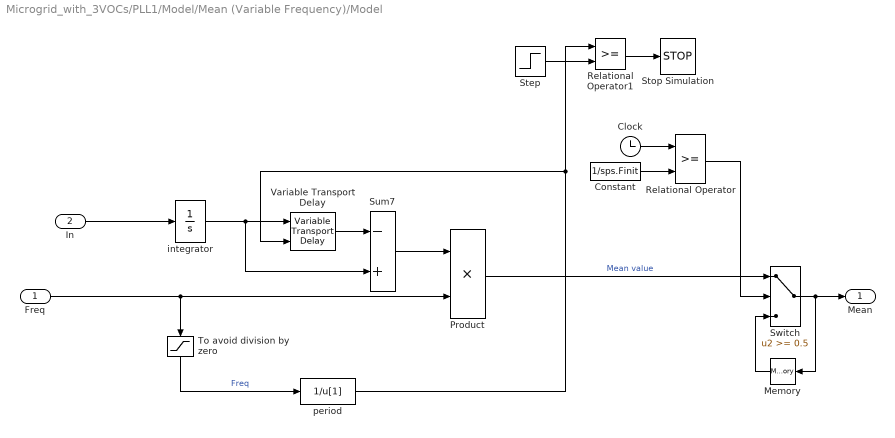
== system Microgrid_with_3VOCs/PLL1/Model/Mean (Variable Frequency)/Model ==
  Freq : Inport  PortDimensions=1
  In : Inport  Port=2
  Clock : Clock
  Constant : Constant  Value=1/sps.Finit
  Memory : Memory  InitialCondition=sps.Vinit
  Product : Product  SaturateOnIntegerOverflow=on  InputSameDT=on  OutDataTypeStr=Inherit: Same as first input
  Relational Operator : RelationalOperator  OutDataTypeStr=boolean  SampleTime=Ts  RndMeth=Nearest
  Relational Operator1 : RelationalOperator  OutDataTypeStr=boolean  RndMeth=Simplest
  Step : Step  Time=0.1  Before=10e6  After=0.016  SampleTime=0
  Stop Simulation : Stop
  Sum7 : Sum  Inputs=-+  SaturateOnIntegerOverflow=on  InputSameDT=on  OutDataTypeStr=Inherit: Same as first input
  Switch : Switch  Threshold=0.5  InputSameDT=on
  To avoid division by zero : Saturate  UpperLimit=1e6  LowerLimit=eps
  Variable Transport Delay : VariableTransportDelay  VariableDelayType=Variable transport delay  MaximumDelay=1/sps.Fmin+eps  MaximumPoints=2048*4  PadeOrder=2
  integrator : Integrator
  period : Fcn  Expr=1/u[1]
  Mean : Outport
  wires:
  Constant/1 -> Relational Operator/2
  To avoid division by zero/1 -> period/1  "Freq"
  Switch/1 -> Memory/1, Mean/1
  Freq/1 -> To avoid division by zero/1, Product/2
  integrator/1 -> Variable Transport Delay/1, Sum7/2
  Sum7/1 -> Product/1
  Variable Transport Delay/1 -> Sum7/1
  Product/1 -> Switch/1  "Mean value"
  In/1 -> integrator/1
  Clock/1 -> Relational Operator/1
  Memory/1 -> Switch/3
  Relational Operator/1 -> Switch/2
  Relational Operator1/1 -> Stop Simulation/1
  Step/1 -> Relational Operator1/2
  period/1 -> Variable Transport Delay/2, Relational Operator1/1

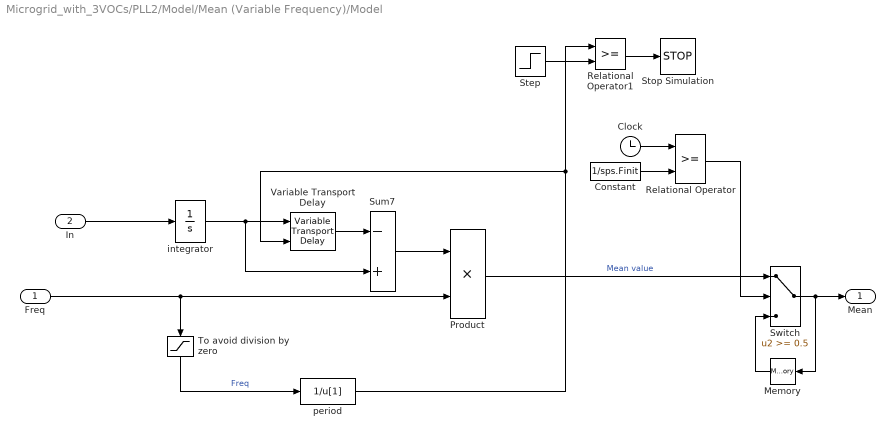
== system Microgrid_with_3VOCs/PLL2/Model/Mean (Variable Frequency)/Model ==
  Freq : Inport  PortDimensions=1
  In : Inport  Port=2
  Clock : Clock
  Constant : Constant  Value=1/sps.Finit
  Memory : Memory  InitialCondition=sps.Vinit
  Product : Product  SaturateOnIntegerOverflow=on  InputSameDT=on  OutDataTypeStr=Inherit: Same as first input
  Relational Operator : RelationalOperator  OutDataTypeStr=boolean  SampleTime=Ts  RndMeth=Nearest
  Relational Operator1 : RelationalOperator  OutDataTypeStr=boolean  RndMeth=Simplest
  Step : Step  Time=0.1  Before=10e6  After=0.016  SampleTime=0
  Stop Simulation : Stop
  Sum7 : Sum  Inputs=-+  SaturateOnIntegerOverflow=on  InputSameDT=on  OutDataTypeStr=Inherit: Same as first input
  Switch : Switch  Threshold=0.5  InputSameDT=on
  To avoid division by zero : Saturate  UpperLimit=1e6  LowerLimit=eps
  Variable Transport Delay : VariableTransportDelay  VariableDelayType=Variable transport delay  MaximumDelay=1/sps.Fmin+eps  MaximumPoints=2048*4  PadeOrder=2
  integrator : Integrator
  period : Fcn  Expr=1/u[1]
  Mean : Outport
  wires:
  Constant/1 -> Relational Operator/2
  To avoid division by zero/1 -> period/1  "Freq"
  Switch/1 -> Memory/1, Mean/1
  Freq/1 -> To avoid division by zero/1, Product/2
  integrator/1 -> Variable Transport Delay/1, Sum7/2
  Sum7/1 -> Product/1
  Variable Transport Delay/1 -> Sum7/1
  Product/1 -> Switch/1  "Mean value"
  In/1 -> integrator/1
  Clock/1 -> Relational Operator/1
  Memory/1 -> Switch/3
  Relational Operator/1 -> Switch/2
  Relational Operator1/1 -> Stop Simulation/1
  Step/1 -> Relational Operator1/2
  period/1 -> Variable Transport Delay/2, Relational Operator1/1

== matlab function Microgrid_with_3VOCs/VoC1/Nonlinearity 1/MATLAB Function ==
  data: V input; I output; Sig input; Phi input
function I = fcn(V,Sig,Phi)

%Piecewise
if V > Phi
    I = Sig * ((2 * Phi) - V);
    
elseif V < -Phi
    I = Sig * ((2 * -Phi) - V);
    
else
    I = Sig * V;
    
end

== matlab function Microgrid_with_3VOCs/VoC/Nonlinearity 1/MATLAB Function ==
  data: V input; I output; Sig input; Phi input
function I = fcn(V,Sig,Phi)

%Piecewise
if V > Phi
    I = Sig * ((2 * Phi) - V);
    
elseif V < -Phi
    I = Sig * ((2 * -Phi) - V);
    
else
    I = Sig * V;
    
end

== matlab function Microgrid_with_3VOCs/VoC2/Nonlinearity 1/MATLAB Function ==
  data: V input; I output; Sig input; Phi input
function I = fcn(V,Sig,Phi)

%Piecewise
if V > Phi
    I = Sig * ((2 * Phi) - V);
    
elseif V < -Phi
    I = Sig * ((2 * -Phi) - V);
    
else
    I = Sig * V;
    
end
